simulink model "RosSimulink"  (R2025b)
settings: Solver=FixedStepDiscrete  StartTime=0.0  StopTime=200  FixedStep=0.01  RelTol=1e-3
model workspace (MAT data in the model file):
  firstWarning = 1
  originalScenarioChecksum = '24A1F6683B00076D3D3B9ECE58E87B1E'
values from neighbouring files (symbols this model uses):
  data =     [TrafficLight_drivingscenario.mat]
undefined symbols (not defined in the file or in its folder): data_SL_Info, DiscIntNeverNeededParam
libraries: ros2lib x3, simulink x1
settings Model: Creator=maric  LastModifiedBy=maric

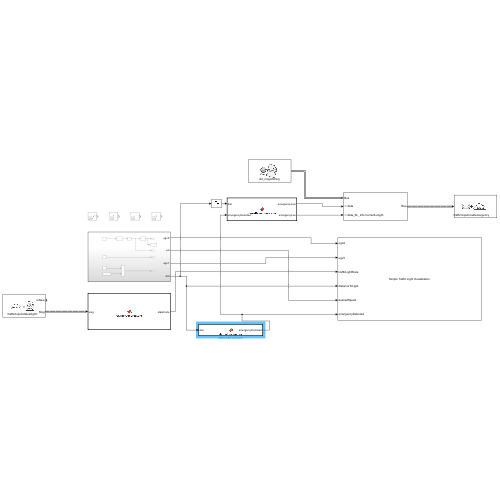
[thumbnail: Simulink's stored preview of the top-level diagram]
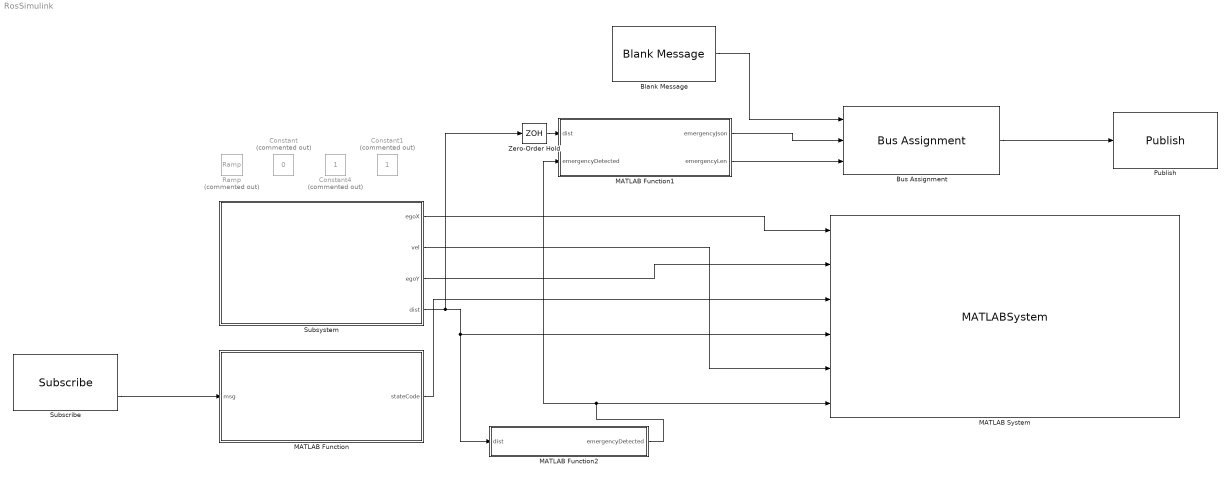
== system RosSimulink ==
  Blank Message : ros2lib/Blank Message  messageClass=Message  entityType=std_msgs/String  messageType=std_msgs/String  SampleTime=inf
  Bus Assignment : BusAssignment  AssignedSignals=data,data_SL_Info.CurrentLength
  Constant : Constant  Commented=on  Value=0
  Constant1 : Constant  Commented=on
  Constant4 : Constant  Commented=on
  MATLAB Function : MATLAB Function  TreatAsAtomicUnit=on
  MATLAB Function1 : MATLAB Function  TreatAsAtomicUnit=on
  MATLAB Function2 : MATLAB Function  TreatAsAtomicUnit=on
  MATLAB System : MATLABSystem  System=SimpleTrafficLightScenario  Ts=0.01  RoadLength=200  RoadWidth=4  TrafficLightX=100  TrafficLightY=-2.3  StopLineX=90  LaneWidth=3.5  NumLanes=2  PavementWidth=3  DisableVisualization=off
      mask Type: SimpleTrafficLightScenario
  Publish : ros2lib/Publish  topicSource=Select from ROS network  topic=/traffic/input/road/emergency  messageType=std_msgs/String  QOSHistory=Keep last  QOSDepth=10  QOSReliability=Reliable  QOSDurability=Volatile  QOSDeadline=Inf  QOSLifespan=Inf  QOSLiveliness=Automatic  QOSLeaseDuration=Inf  QOSAvoidROSNamespaceConventions=off
  Ramp : simulink/Sources/Ramp  Commented=on  slope=2  start=0  InitialOutput=0
  Subscribe : ros2lib/Subscribe  topicSource=Select from ROS network  topic=/traffic/input/status/light1  messageType=std_msgs/String  sampleTime=-1  QOSHistory=Keep last  QOSDepth=10  QOSReliability=Reliable  QOSDurability=Volatile  QOSDeadline=Inf  QOSLifespan=Inf  QOSLiveliness=Automatic  QOSLeaseDuration=Inf  QOSAvoidROSNamespaceConventions=off
  Subsystem : Subsystem
  Zero-Order Hold : ZeroOrderHold
  wires:
  MATLAB Function2/1(emergencyDetected) -> MATLAB Function1/2(emergencyDetected), MATLAB System/6
  Subscribe/2 -> MATLAB Function/1(msg)
  MATLAB Function/1(stateCode) -> MATLAB System/3
  Subsystem/1(egoX) -> MATLAB System/1
  Subsystem/3(egoY) -> MATLAB System/2
  Subsystem/2(vel) -> MATLAB System/5
  Subsystem/4(dist) -> MATLAB Function2/1(dist), MATLAB System/4, Zero-Order Hold/1
  Bus Assignment/1 -> Publish/1
  Blank Message/1 -> Bus Assignment/1
  MATLAB Function1/1(emergencyJson) -> Bus Assignment/2
  MATLAB Function1/2(emergencyLen) -> Bus Assignment/3
  Zero-Order Hold/1 -> MATLAB Function1/1(dist)

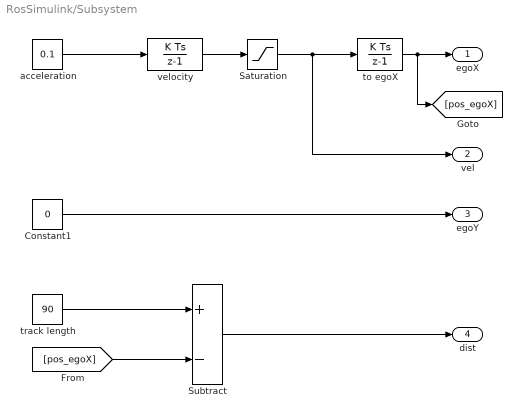
== system RosSimulink/Subsystem ==
  Constant1 : Constant  Value=0
  Saturation : Saturate  UpperLimit=30  LowerLimit=0
  Subtract : Sum  Inputs=+-
  acceleration : Constant  Value=0.1
  to egoX : DiscreteIntegrator  SampleTime=0.01  UpperSaturationLimit=13.9  LowerSaturationLimit=0  ICPrevOutput=DiscIntNeverNeededParam  ICPrevScaledInput=DiscIntNeverNeededParam
  track length : Constant  Value=90
  velocity : DiscreteIntegrator  LimitOutput=on  UpperSaturationLimit=13.9  LowerSaturationLimit=0  ICPrevOutput=DiscIntNeverNeededParam  ICPrevScaledInput=DiscIntNeverNeededParam
  egoX : Outport
  vel : Outport  Port=2
  egoY : Outport  Port=3
  dist : Outport  Port=4
  wires:
  velocity/1 -> Saturation/1
  Saturation/1 -> to egoX/1, vel/1
  Constant1/1 -> egoY/1
  track length/1 -> Subtract/1
  [pos_egoX] -> Subtract/2
  Subtract/1 -> dist/1
  to egoX/1 -> [pos_egoX], egoX/1
  acceleration/1 -> velocity/1

== matlab function RosSimulink/MATLAB Function ==
  data: msg input; stateCode output
function stateCode = extractCurrentState(msg)

% Output:
% 0 = UNKNOWN
% 1 = RED
% 2 = YELLOW
% 3 = GREEN

stateCode = uint8(0);

% Get ROS2 std_msgs/String content
txt = char(msg.data);

% Force it to be one row
txt = reshape(txt, 1, []);

% Remove null characters
txt(txt == char(0)) = ' ';

% Search directly for the traffic light states
if ~isempty(strfind(txt, 'RED'))
    stateCode = uint8(1);

elseif ~isempty(strfind(txt, 'YELLOW'))
    stateCode = uint8(2);

elseif ~isempty(strfind(txt, 'GREEN'))
    stateCode = uint8(3);

else
    stateCode = uint8(0);
end

== matlab function RosSimulink/MATLAB Function2 ==
  data: dist input; emergencyDetected output
function emergencyDetected = detectEmergency(dist)
%#codegen

if dist >= 0 && dist < 60
    emergencyDetected = 1;
else
    emergencyDetected = 0;
end

end

== matlab function RosSimulink/MATLAB Function1 ==
  data: dist input; emergencyJson output; emergencyLen output; emergencyDetected input
function [emergencyJson, emergencyLen] = makeEmergencyJson(dist, emergencyDetected)
%#codegen

MAX_LEN = 128;

emergencyJson = zeros(1, MAX_LEN, 'uint8');

if emergencyDetected ~= 0
    emergencyText = 'true';
else
    emergencyText = 'false';
end

temp = sprintf(['{"emergency_present":%s,' ...
                '"type":"ambulance",' ...
                '"id":"emg_01",' ...
                '"pos":%.2f,' ...
                '"speed":1.20,' ...
                '"siren":%s}'], ...
                emergencyText, ...
                dist, ...
                emergencyText);

n = min(length(temp), MAX_LEN);

for i = 1:n
    emergencyJson(i) = uint8(temp(i));
end

emergencyLen = uint32(n);

end
